simulink model "Systems_Task1_1"  (R2022a)
settings: Solver=VariableStepAuto  StartTime=0.0  StopTime=10000  RelTol=1e-3
settings Model: Creator=Joel  LastModifiedBy=Joel

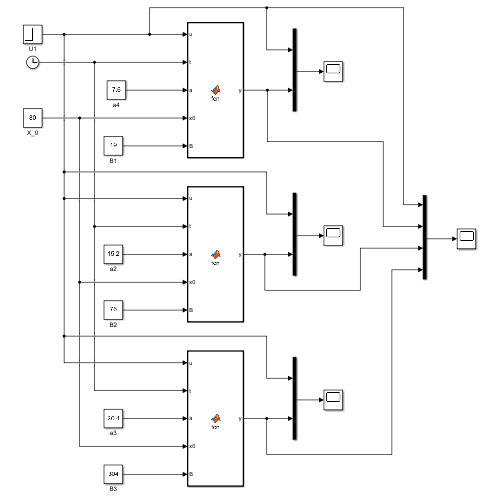
[thumbnail: Simulink's stored preview of the top-level diagram]
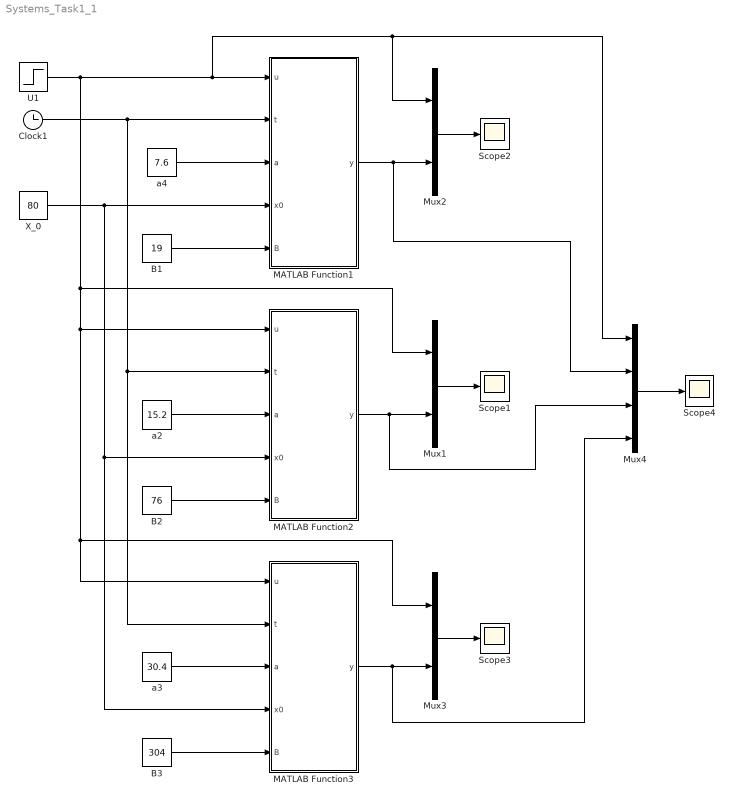
== system Systems_Task1_1 ==
  B1 : Constant  Value=19
  B2 : Constant  Value=76
  B3 : Constant  Value=304
  Clock1 : Clock
  MATLAB Function1 : MATLAB Function  TreatAsAtomicUnit=on
  MATLAB Function2 : MATLAB Function  TreatAsAtomicUnit=on
  MATLAB Function3 : MATLAB Function  TreatAsAtomicUnit=on
  Mux1 : Mux  Inputs=2
  Mux2 : Mux  Inputs=2
  Mux3 : Mux  Inputs=2
  Mux4 : Mux
  Scope{1..4} (4 alike) : Scope
  U1 : Step  Time=100  Before=76  After=200  SampleTime=0
  X_0 : Constant  Value=80
  a2 : Constant  Value=15.2
  a3 : Constant  Value=30.4
  a4 : Constant  Value=7.6
  wires:
  MATLAB Function1/1(y) -> Mux4/2, Mux2/2
  Mux2/1 -> Scope2/1
  B1/1 -> MATLAB Function1/5(B)
  B2/1 -> MATLAB Function2/5(B)
  Mux1/1 -> Scope1/1
  a2/1 -> MATLAB Function2/3(a)
  MATLAB Function2/1(y) -> Mux4/3, Mux1/2
  MATLAB Function3/1(y) -> Mux4/4, Mux3/2
  X_0/1 -> MATLAB Function1/4(x0), MATLAB Function3/4(x0), MATLAB Function2/4(x0)
  a3/1 -> MATLAB Function3/3(a)
  Clock1/1 -> MATLAB Function1/2(t), MATLAB Function3/2(t), MATLAB Function2/2(t)
  Mux3/1 -> Scope3/1
  U1/1 -> Mux2/1, Mux4/1, MATLAB Function1/1(u), Mux1/1, MATLAB Function2/1(u), Mux3/1, MATLAB Function3/1(u)
  B3/1 -> MATLAB Function3/5(B)
  a4/1 -> MATLAB Function1/3(a)
  Mux4/1 -> Scope4/1

== matlab function Systems_Task1_1/MATLAB Function1 ==
  data: u input; t input; a input; x0 input; y output; B input
function y = fcn(u, t, a, x0, B)

A = x0*a -B-u;
y = (A*exp(-a*t/2560)+u+B)/a;

== matlab function Systems_Task1_1/MATLAB Function2 ==
  data: u input; t input; a input; x0 input; y output; B input
function y = fcn(u, t, a, x0, B)

A = x0*a -B-u;
y = (A*exp(-a*t/2560)+u+B)/a;

== matlab function Systems_Task1_1/MATLAB Function3 ==
  data: u input; t input; a input; x0 input; y output; B input
function y = fcn(u, t, a, x0, B)

A = x0*a -B-u;
y = (A*exp(-a*t/2560)+u+B)/a;
